simulink model "S_C"  (R2013a)
settings: Solver=ode45  StartTime=0.0  StopTime=0.2  RelTol=1e-3
settings Model: Creator=MEHEDI HASSAN  LastModifiedBy=BORAT
settings OptimizationCC: InlineParams=on
settings DebuggingCC: SolverPrmCheckMsg=none  ModelReferenceExtraNoncontSigs=none

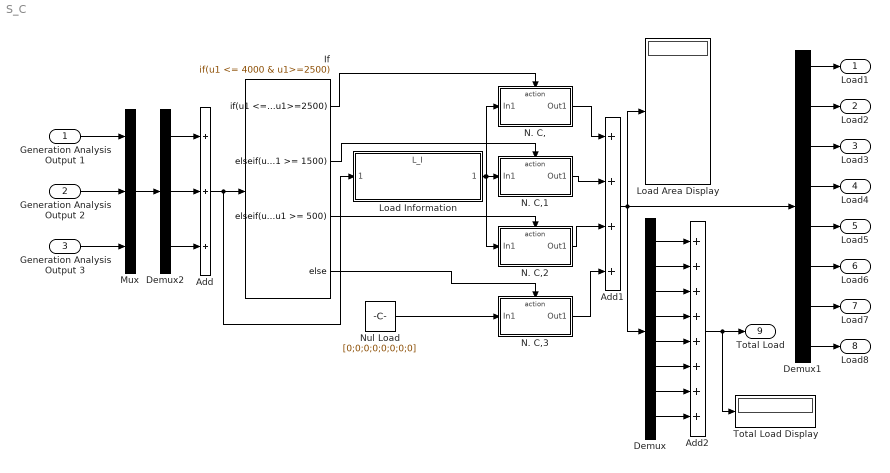
== system S_C ==
  Generation Analysis Output 1 : Inport
  Generation Analysis Output 2 : Inport  Port=2
  Generation Analysis Output 3 : Inport  Port=3
  Add : Sum  Inputs=+++
  Add1 : Sum  Inputs=++++
  Add2 : Sum  Inputs=++++++++
  Demux : Demux  Outputs=8
  Demux1 : Demux  Outputs=8
  Demux2 : Demux  Outputs=3
  If : If  IfExpression=u1 <= 4000 & u1>=2500  ElseIfExpressions=u1 < 2500 & u1 >= 1500, u1 < 1500 & u1 >= 500
  Load Area Display : Display
  Load Information : ModelReference  ModelNameDialog=L_I.slx  SimulationMode=Normal  ModelReferenceVersion=1.7  CopyOfModelName=L_I.slx  DefaultDataLogging=on
  Mux : Mux  Inputs=3
  N. C, : Subsystem  TreatAsAtomicUnit=on
  N. C,1 : Subsystem  TreatAsAtomicUnit=on
  N. C,2 : Subsystem  TreatAsAtomicUnit=on
  N. C,3 : Subsystem  TreatAsAtomicUnit=on
  Nul Load : Constant  Value=[0;0;0;0;0;0;0;0]
  Total Load Display : Display
  Load1 : Outport
  Load2 : Outport  Port=2
  Load3 : Outport  Port=3
  Load4 : Outport  Port=4
  Load5 : Outport  Port=5
  Load6 : Outport  Port=6
  Load7 : Outport  Port=7
  Load8 : Outport  Port=8
  Total Load : Outport  Port=9
  wires:
  Nul Load/1 -> N. C,3/1(In1)
  If/1 -> N. C,/Action
  If/2 -> N. C,1/Action
  If/3 -> N. C,2/Action
  If/4 -> N. C,3/Action
  Load Information/1 -> N. C,2/1(In1), N. C,/1(In1), N. C,1/1(In1)
  N. C,/1(Out1) -> Add1/1
  N. C,1/1(Out1) -> Add1/2
  N. C,2/1(Out1) -> Add1/3
  N. C,3/1(Out1) -> Add1/4
  Demux/1 -> Add2/1
  Demux/2 -> Add2/2
  Demux/3 -> Add2/3
  Demux/4 -> Add2/4
  Demux/5 -> Add2/5
  Demux/6 -> Add2/6
  Demux/7 -> Add2/7
  Demux/8 -> Add2/8
  Add1/1 -> Demux1/1, Demux/1, Load Area Display/1
  Add2/1 -> Total Load/1, Total Load Display/1
  Demux1/1 -> Load1/1
  Demux1/2 -> Load2/1
  Demux1/3 -> Load3/1
  Demux1/4 -> Load4/1
  Demux1/5 -> Load5/1
  Demux1/6 -> Load6/1
  Demux1/7 -> Load7/1
  Demux1/8 -> Load8/1
  Generation Analysis Output 1/1 -> Mux/1
  Generation Analysis Output 2/1 -> Mux/2
  Generation Analysis Output 3/1 -> Mux/3
  Mux/1 -> Demux2/1
  Add/1 -> If/1, Load Information/1
  Demux2/1 -> Add/1
  Demux2/2 -> Add/2
  Demux2/3 -> Add/3

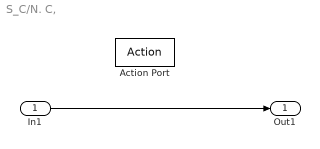
== system S_C/N. C, ==
  In1 : Inport
  Action Port : ActionPort  ActionType=then
  Out1 : Outport
  wires:
  In1/1 -> Out1/1

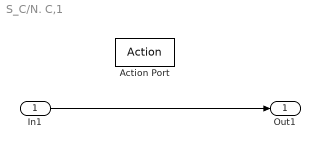
== system S_C/N. C,1 ==
  In1 : Inport
  Action Port : ActionPort  ActionType=elseif
  Out1 : Outport
  wires:
  In1/1 -> Out1/1

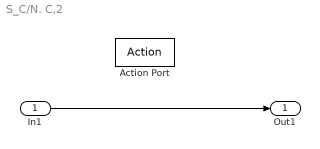
== system S_C/N. C,2 ==
  In1 : Inport
  Action Port : ActionPort  ActionType=elseif
  Out1 : Outport
  wires:
  In1/1 -> Out1/1

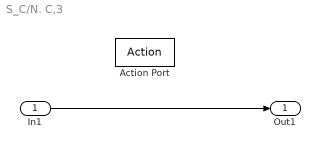
== system S_C/N. C,3 ==
  In1 : Inport
  Action Port : ActionPort  ActionType=else
  Out1 : Outport
  wires:
  In1/1 -> Out1/1
